simulink model "SHsimplify"  (R2013a)
settings: Solver=ode45  StartTime=0.0  StopTime=20  RelTol=1e-3
settings Model: Creator=mainster  LastModifiedBy=mainster

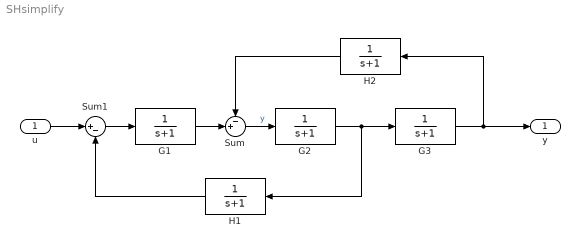
== system SHsimplify ==
  u : Inport
  G1 : TransferFcn  Denominator=[1 1]
  G2 : TransferFcn  Denominator=[1 1]
  G3 : TransferFcn  Denominator=[1 1]
  H1 : TransferFcn  Denominator=[1 1]
  H2 : TransferFcn  Denominator=[1 1]
  Sum : Sum  Inputs=-+|
  Sum1 : Sum  Inputs=|+-
  y : Outport
  wires:
  u/1 -> Sum1/1
  Sum1/1 -> G1/1
  Sum/1 -> G2/1  "y"
  G2/1 -> H1/1, G3/1
  H2/1 -> Sum/1
  G1/1 -> Sum/2
  H1/1 -> Sum1/2
  G3/1 -> H2/1, y/1
